simulink model "untitled"  (R2021a)
settings: Solver=FixedStepAuto  StartTime=0.0  StopTime=0.1  FixedStep=1e-3  RelTol=1e-3
undefined symbols (not defined in the file or in its folder): kd, ki, kp
settings Model: Creator=Saniya  LastModifiedBy=Saniya

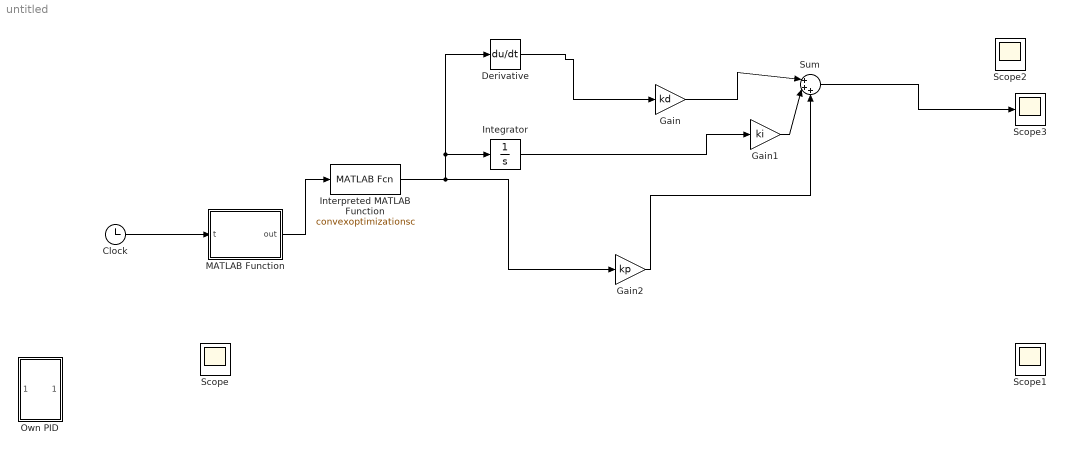
== system untitled ==
  Clock : Clock
  Derivative : Derivative
  Gain : Gain  Gain=kd
  Gain1 : Gain  Gain=ki
  Gain2 : Gain  Gain=kp
  Integrator : Integrator
  Interpreted MATLAB Function : MATLABFcn  MATLABFcn=convexoptimizationsc  OutputDimensions=2  Output1D=off
  MATLAB Function : MATLAB Function  TreatAsAtomicUnit=on
  Own PID : Subsystem
  Scope{,1..3} (4 alike) : Scope
  Sum : Sum  Inputs=|+++
  wires:
  MATLAB Function/1(out) -> Interpreted MATLAB Function/1
  Clock/1 -> MATLAB Function/1(t)
  Sum/1 -> Scope3/1
  Gain1/1 -> Sum/2
  Integrator/1 -> Gain1/1
  Gain/1 -> Sum/1
  Derivative/1 -> Gain/1
  Interpreted MATLAB Function/1 -> Integrator/1, Derivative/1, Gain2/1
  Gain2/1 -> Sum/3

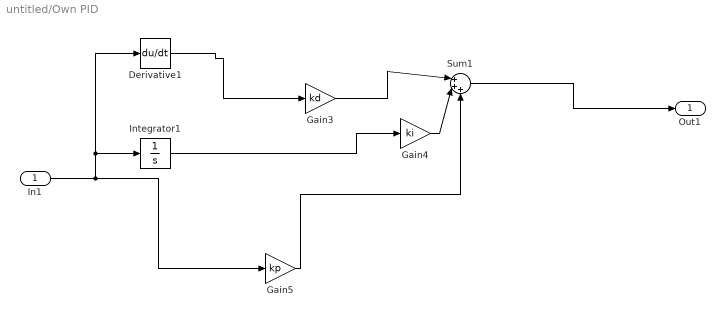
== system untitled/Own PID ==
  In1 : Inport
  Derivative1 : Derivative
  Gain3 : Gain  Gain=kd
  Gain4 : Gain  Gain=ki
  Gain5 : Gain  Gain=kp
  Integrator1 : Integrator
  Sum1 : Sum  Inputs=|+++
  Out1 : Outport
  wires:
  Gain5/1 -> Sum1/3
  Gain4/1 -> Sum1/2
  Integrator1/1 -> Gain4/1
  In1/1 -> Integrator1/1, Derivative1/1, Gain5/1
  Derivative1/1 -> Gain3/1
  Gain3/1 -> Sum1/1
  Sum1/1 -> Out1/1

== matlab function untitled/MATLAB Function ==
  data: out output; t input
function out = fcn(t)
h=t.*eye(3,12);
h_dot=t.*eye(3,12);
V=eig(transpose(h)*h);
%V=t.*eye(12,12);
out = [h;h_dot;V];
end
